simulink model "fir16tap"  (Simulink 10.0)
settings: Solver=FixedStepDiscrete  StartTime=0.0  StopTime=3000  RelTol=1e-3
settings Model: Creator=moeller  LastModifiedBy=bhisma
settings DataIOCC: LimitDataPoints=on  SignalLoggingSaveFormat=ModelDataLogs
settings OptimizationCC: BlockReduction=off  ConditionallyExecuteInputs=off  ExpressionDepthLimit=2147483647
settings DebuggingCC: SolverPrmCheckMsg=warning  MultiTaskCondExecSysMsg=warning  SingleTaskRateTransMsg=error  FcnCallInpInsideContextMsg=warning  StateNameClashWarn=warning
settings GRTTargetCC: GeneratePreprocessorConditionals=Disable all
settings ConfigComp: CovExternalEMLEnable=off  CovSFcnEnable=off

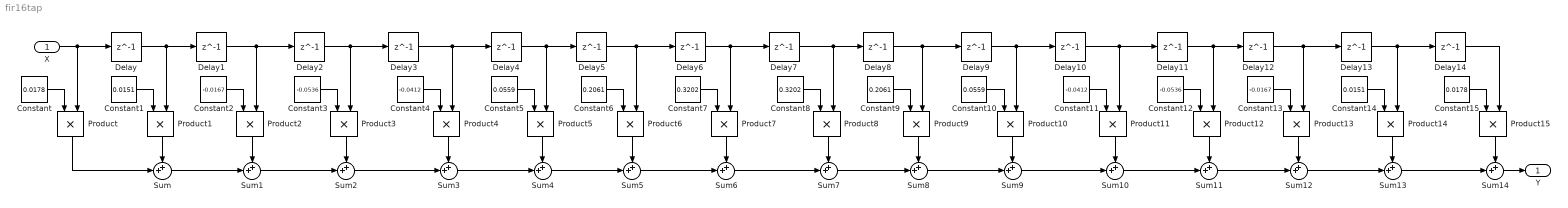
== system fir16tap ==
  X : Inport
  Constant : Constant  Value=0.0178  OutDataTypeStr=Inherit: Inherit via back propagation
  Constant1 : Constant  Value=0.0151  OutDataTypeStr=Inherit: Inherit via back propagation
  Constant10 : Constant  Value=0.0559  OutDataTypeStr=Inherit: Inherit via back propagation
  Constant11 : Constant  Value=-0.0412  OutDataTypeStr=Inherit: Inherit via back propagation
  Constant12 : Constant  Value=-0.0536  OutDataTypeStr=Inherit: Inherit via back propagation
  Constant13 : Constant  Value=-0.0167  OutDataTypeStr=Inherit: Inherit via back propagation
  Constant14 : Constant  Value=0.0151  OutDataTypeStr=Inherit: Inherit via back propagation
  Constant15 : Constant  Value=0.0178  OutDataTypeStr=Inherit: Inherit via back propagation
  Constant2 : Constant  Value=-0.0167  OutDataTypeStr=Inherit: Inherit via back propagation
  Constant3 : Constant  Value=-0.0536  OutDataTypeStr=Inherit: Inherit via back propagation
  Constant4 : Constant  Value=-0.0412  OutDataTypeStr=Inherit: Inherit via back propagation
  Constant5 : Constant  Value=0.0559  OutDataTypeStr=Inherit: Inherit via back propagation
  Constant6 : Constant  Value=0.2061  OutDataTypeStr=Inherit: Inherit via back propagation
  Constant7 : Constant  Value=0.3202  OutDataTypeStr=Inherit: Inherit via back propagation
  Constant8 : Constant  Value=0.3202  OutDataTypeStr=Inherit: Inherit via back propagation
  Constant9 : Constant  Value=0.2061  OutDataTypeStr=Inherit: Inherit via back propagation
  Delay{,1..14} (15 alike) : Delay  DelayLength=1  SampleTime=1
  Product{,1..15} (16 alike) : Product  OutDataTypeStr=fixdt(1,32,16)  RndMeth=Zero
  Sum{,1..14} (15 alike) : Sum  Inputs=++|  AccumDataTypeStr=fixdt(1,32,16)  OutDataTypeStr=fixdt(1,32,16)
  Y : Outport
  wires:
  X/1 -> Delay/1, Product/2
  Constant/1 -> Product/1
  Product/1 -> Sum/2
  Constant1/1 -> Product1/1
  Product1/1 -> Sum/1
  Delay/1 -> Delay1/1, Product1/2
  Constant2/1 -> Product2/1
  Delay1/1 -> Delay2/1, Product2/2
  Constant3/1 -> Product3/1
  Delay2/1 -> Product3/2, Delay3/1
  Product2/1 -> Sum1/1
  Sum/1 -> Sum1/2
  Sum1/1 -> Sum2/2
  Product3/1 -> Sum2/1
  Sum2/1 -> Sum3/2
  Product4/1 -> Sum3/1
  Constant4/1 -> Product4/1
  Delay3/1 -> Product4/2, Delay4/1
  Constant5/1 -> Product5/1
  Product5/1 -> Sum4/1
  Delay4/1 -> Delay5/1, Product5/2
  Constant6/1 -> Product6/1
  Delay5/1 -> Delay6/1, Product6/2
  Constant7/1 -> Product7/1
  Delay6/1 -> Product7/2, Delay7/1
  Product6/1 -> Sum5/1
  Sum4/1 -> Sum5/2
  Sum5/1 -> Sum6/2
  Product7/1 -> Sum6/1
  Sum6/1 -> Sum7/2
  Product8/1 -> Sum7/1
  Constant8/1 -> Product8/1
  Delay7/1 -> Product8/2, Delay8/1
  Sum3/1 -> Sum4/2
  Constant9/1 -> Product9/1
  Delay8/1 -> Delay9/1, Product9/2
  Constant10/1 -> Product10/1
  Delay9/1 -> Product10/2, Delay10/1
  Product9/1 -> Sum8/1
  Sum7/1 -> Sum8/2
  Sum8/1 -> Sum9/2
  Product10/1 -> Sum9/1
  Sum9/1 -> Sum10/2
  Product11/1 -> Sum10/1
  Constant11/1 -> Product11/1
  Delay10/1 -> Product11/2, Delay11/1
  Constant12/1 -> Product12/1
  Product12/1 -> Sum11/1
  Delay11/1 -> Delay12/1, Product12/2
  Constant13/1 -> Product13/1
  Delay12/1 -> Delay13/1, Product13/2
  Constant14/1 -> Product14/1
  Delay13/1 -> Product14/2, Delay14/1
  Product13/1 -> Sum12/1
  Sum11/1 -> Sum12/2
  Sum12/1 -> Sum13/2
  Product14/1 -> Sum13/1
  Sum13/1 -> Sum14/2
  Product15/1 -> Sum14/1
  Constant15/1 -> Product15/1
  Delay14/1 -> Product15/2
  Sum10/1 -> Sum11/2
  Sum14/1 -> Y/1
